simulink model "algorithm"  (R2023a)
settings: Solver=VariableStepAuto  StartTime=0.0  StopTime=10.0  RelTol=1e-3
settings Model: Creator=fercl  LastModifiedBy=fercl

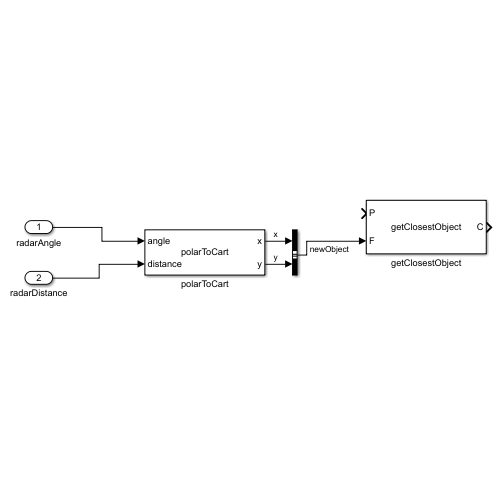
[thumbnail: Simulink's stored preview of the top-level diagram]
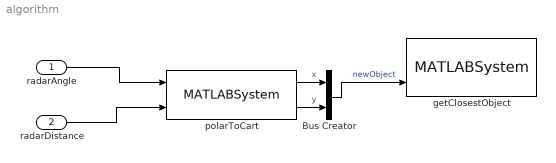
== system algorithm ==
  radarAngle : Inport
  radarDistance : Inport  Port=2
  Bus Creator : BusCreator  Inputs=2
  getClosestObject : MATLABSystem  System=getClosestObject  SimulateUsing=Code generation
      mask Type: getClosestObject
      mask Display:
      | disp('getClosestObject');
      | port_label('input',1,'P');
      | port_label('input',2,'F');
      | port_label('output',1,'C');
  polarToCart : MATLABSystem  System=polarToCart  SimulateUsing=Code generation
      mask Type: polarToCart
      mask Display:
      | disp('polarToCart');
      | port_label('input',1,'angle');
      | port_label('input',2,'distance');
      | port_label('output',1,'x');
      | port_label('output',2,'y');
  wires:
  radarAngle/1 -> polarToCart/1
  radarDistance/1 -> polarToCart/2
  polarToCart/2 -> Bus Creator/2  "y"
  polarToCart/1 -> Bus Creator/1  "x"
  Bus Creator/1 -> getClosestObject/2  "newObject"
